simulink subsystem "Simple_State_Observer"  (R2024b)
settings: Solver=VariableStepAuto  StartTime=0.0  StopTime=10.0  RelTol=1e-3
undefined symbols (not defined in the file or in its folder): degs2rpm, H1
settings Model: Creator=Riccardo Grosso  LastModifiedBy=Buton

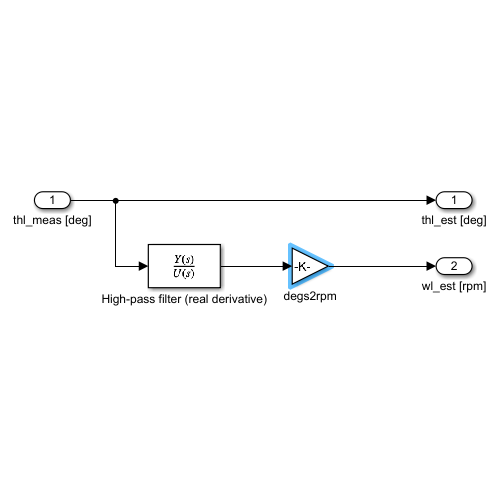
[thumbnail: Simulink's stored preview of the top-level diagram]
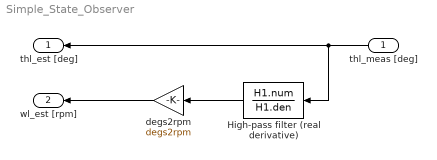
== system Simple_State_Observer ==
  thl_meas [deg] : Inport
  High-pass filter (real derivative) : TransferFcn  Numerator=H1.num  Denominator=H1.den
  degs2rpm : Gain  Gain=degs2rpm
  thl_est [deg] : Outport
  wl_est [rpm] : Outport  Port=2
  wires:
  thl_meas [deg]/1 -> High-pass filter (real derivative)/1, thl_est [deg]/1
  High-pass filter (real derivative)/1 -> degs2rpm/1
  degs2rpm/1 -> wl_est [rpm]/1
